simulink subsystem "Subsystem_Driver_Controllers_BAv01"  (R2022b)
settings: Solver=VariableStepAuto  StartTime=0.0  StopTime=10.0  RelTol=1e-3
undefined symbols (not defined in the file): param
libraries: slpidlib x2
settings Model: Creator=giaco  LastModifiedBy=giaco

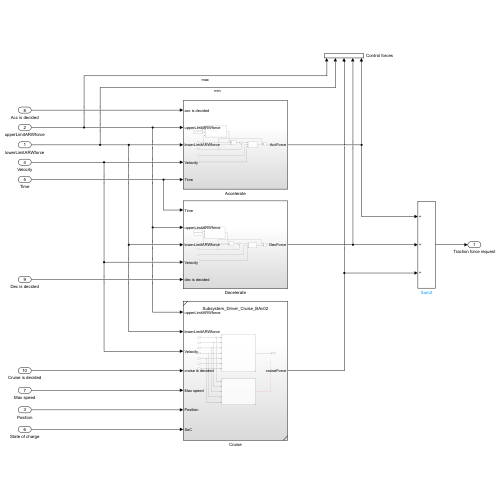
[thumbnail: Simulink's stored preview of the top-level diagram]
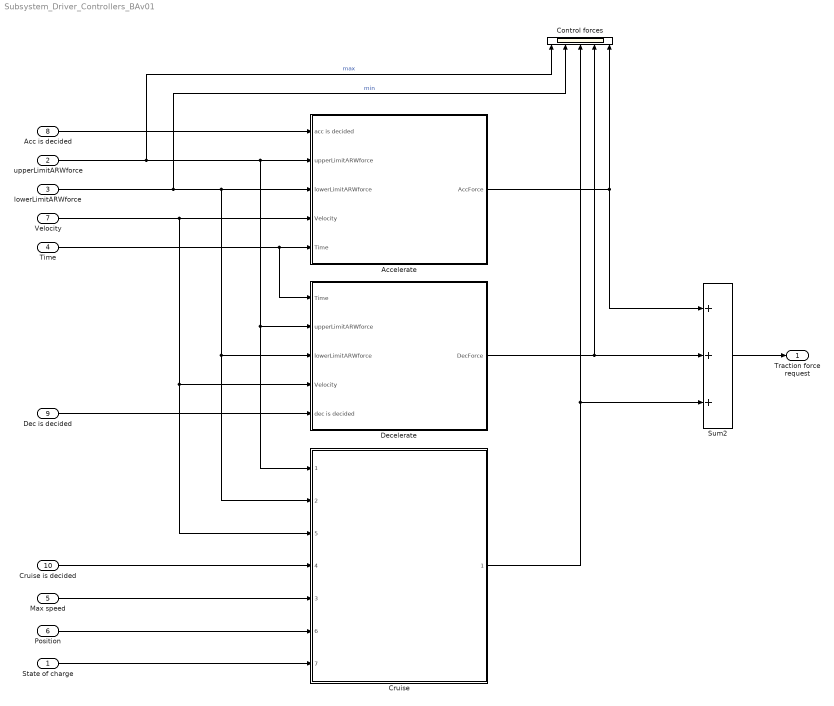
== system Subsystem_Driver_Controllers_BAv01 ==
  State of charge : Inport
  upperLimitARWforce : Inport  Port=2
  lowerLimitARWforce : Inport  Port=3
  Time : Inport  Port=4
  Max speed : Inport  Port=5
  Position : Inport  Port=6
  Velocity : Inport  Port=7
  Acc is decided : Inport  Port=8
  Dec is decided : Inport  Port=9
  Cruise is decided : Inport  Port=10
  Accelerate : Subsystem
  Control forces : Scope  NumInputPorts=5
  Cruise : Subsystem  ReferencedSubsystem=Subsystem_Driver_Cruise_BAv02
      settings: PortSchema="{\"entries\":[{\"content\":{\"sides\":[{\"content\":{\"connectorIds\":[\"In1\",\"In2\",\"In5\",\"In4\",\"In3\",\"In6\",\"In7\"]},\"type\":\"ConnectorPlacement.EquallySpacedRectSide\",\"uuid\":\"ef64809f-0964-4d4c-8634-68fa8e631720\"},{\"content\":{\"connectorIds\":[\"Out1\"],\"side\":\"RIGHT\"},\"type\":\"ConnectorPlacement.EquallySpacedRectSide\",\"uuid\":\"1cbe557a-e7d2-4fe5-a45b-503b50ba40bd\"},{\"content\":{\"connectorIds\":[],\"side\":\"TOP\"},\"type\":\"ConnectorPlacement.EquallySpacedRectSide\",\"uuid\":\"3b2eda76-9c7f-491f-ad4d-397cb13a64b5\"}]},\"type\":\"ConnectorPlacement.EquallySpacedConnector\",\"uuid\":\"83c1d113-dee0-4e25-92c9-f13a92a06a93\"}],\"packageUris\":[\"http://schema.mathworks.com/mf0/Connector/R2020b\"],\"version\":\"1.0\"}"
  Decelerate : Subsystem
  Sum2 : Sum  Inputs=+++
  Traction force request : Outport
  wires:
  upperLimitARWforce/1 -> Control forces/1, Accelerate/2(upperLimitARWforce), Decelerate/2(upperLimitARWforce), Cruise/1  "max"
  Max speed/1 -> Cruise/3
  Acc is decided/1 -> Accelerate/1(acc is decided)
  Accelerate/1(AccForce) -> Control forces/5, Sum2/1
  lowerLimitARWforce/1 -> Accelerate/3(lowerLimitARWforce), Decelerate/3(lowerLimitARWforce), Cruise/2, Control forces/2  "min"
  Sum2/1 -> Traction force request/1
  Decelerate/1(DecForce) -> Sum2/2, Control forces/4
  Time/1 -> Accelerate/5(Time), Decelerate/1(Time)
  State of charge/1 -> Cruise/7
  Dec is decided/1 -> Decelerate/5(dec is decided)
  Cruise/1 -> Control forces/3, Sum2/3
  Position/1 -> Cruise/6
  Cruise is decided/1 -> Cruise/4
  Velocity/1 -> Accelerate/4(Velocity), Decelerate/4(Velocity), Cruise/5

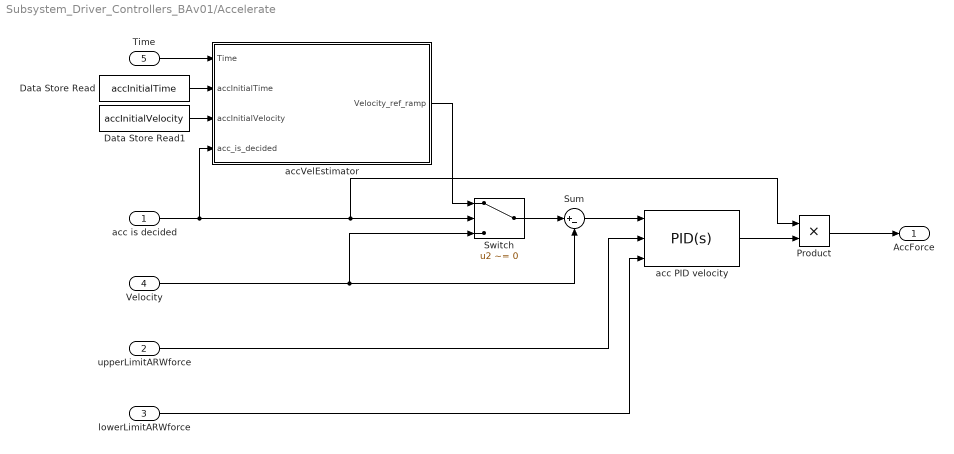
== system Subsystem_Driver_Controllers_BAv01/Accelerate ==
  acc is decided : Inport
  upperLimitARWforce : Inport  Port=2
  lowerLimitARWforce : Inport  Port=3
  Velocity : Inport  Port=4
  Time : Inport  Port=5
  Data Store Read : DataStoreRead  DataStoreName=accInitialTime  IndexOptions=Index vector (dialog)  Indices=1  OutputSizes=1
  Data Store Read1 : DataStoreRead  DataStoreName=accInitialVelocity  IndexOptions=Index vector (dialog)  Indices=1  OutputSizes=1
  Product : Product
  Sum : Sum  Inputs=|+-
  Switch : Switch  Criteria=u2 ~= 0  SaturateOnIntegerOverflow=off  InputSameDT=off
  acc PID velocity : slpidlib/PID Controller  Controller=PID  Form=Ideal  TimeDomain=Continuous-time  UseExternalTs=off  SampleTime=-1  IntegratorMethod=Forward Euler  FilterMethod=Forward Euler  ControllerParametersSource=internal  P=4000  I=1/(1/80)  UseKiTs=off  D=0  N=100  UseFilter=on  TunerSelectOption=Transfer Function Based (PID Tuner App)  InitialConditionSource=internal  InitialConditionForIntegrator=0  InitialConditionForFilter=0  DifferentiatorICPrevScaledInput=0  ExternalReset=none  TrackingMode=off  Kt=1  LimitOutput=on  SatLimitsSource=external  UpperSaturationLimit=param.motor.maxTorque * param.motor.transmissionRatio / param.suspension.wheelRadius  LowerSaturationLimit=param.motor.minTorque * param.motor.transmissionRatio / param.suspension.wheelRadius  LinearizeAsGain=on  AntiWindupMode=clamping  Kb=1  LimitIntegrator=off  UpperIntegratorSaturationLimit=inf  LowerIntegratorSaturationLimit=-inf  POutMin=[]  POutMax=[]  IOutMin=[]  IOutMax=[]  DOutMin=[]  DOutMax=[]  NOutMin=[]  NOutMax=[]  SumOutMin=[]  SumOutMax=[]  SaturationOutMin=[]  SaturationOutMax=[]  PParamMin=[]  PParamMax=[]  IParamMin=[]  IParamMax=[]  DParamMin=[]  DParamMax=[]  NParamMin=[]  NParamMax=[]  KbParamMin=[]  KbParamMax=[]  KtParamMin=[]  KtParamMax=[]  KbOutMin=[]  KbOutMax=[]  KtOutMin=[]  KtOutMax=[]  IntegratorOutMin=[]  IntegratorOutMax=[]  FilterOutMin=[]  FilterOutMax=[]  SumI1OutMin=[]  SumI1OutMax=[]  SumI2OutMin=[]  SumI2OutMax=[]  SumI3OutMin=[]  SumI3OutMax=[]  SumI4OutMin=[]  SumI4OutMax=[]  SumDOutMin=[]  SumDOutMax=[]  DifferentiatorOutMin=[]  DifferentiatorOutMax=[]  FilterDiffOutCoefMin=[]  FilterDiffOutCoefMax=[]  ReciprocalOutMin=[]  ReciprocalOutMax=[]  SumDenOutMin=[]  SumDenOutMax=[]  SumNumOutMin=[]  SumNumOutMax=[]  DivideOutMin=[]  DivideOutMax=[]  UdiffTsProdOutMin=[]  UdiffTsProdOutMax=[]  NTsProdOutMin=[]  NTsProdOutMax=[]  UintegralTsProdOutMin=[]  UintegralTsProdOutMax=[]  UngainTsProdOutMin=[]  UngainTsProdOutMax=[]  ClampingZeroOutDataTypeStr=Inherit: Inherit via back propagation  ClampingZeroOutMin=[]  ClampingZeroOutMax=[]  FilterDenConstantOutDataTypeStr=Inherit: Inherit via back propagation  FilterDenConstantOutMin=[]  FilterDenConstantOutMax=[]  PCopyOutDataTypeStr=Inherit: Inherit via back propagation  PCopyOutMin=[]  PCopyOutMax=[]  NCopyOutDataTypeStr=Inherit: Inherit via back propagation  NCopyOutMin=[]  NCopyOutMax=[]  IntegratorContinuousStateAttributes=''  IntegratorStateMustResolveToSignalObject=off  IntegratorRTWStateStorageClass=Auto  FilterContinuousStateAttributes=''  FilterStateMustResolveToSignalObject=off  FilterRTWStateStorageClass=Auto  ParallelPVariant=Passthrough  IdealPVariant=InternalParameters  IVariant=InternalParameters  DVariant=InternalParameters  IntegratorVariant=Continuous  SatVariant=External  AWVariant=ContClampingIdeal  PCopyVariant=InternalParamsIdeal  TRVariant=Disabled  FdbkBlocksVariant=Forward  IdealPFdbkVariant=Disabled  SatFdbkVariant=Disabled  DerivativeFilterVariant=ContFilter  NVariant=InternalParameters  NCopyVariant=Disabled  FilterICVariant=InternalICsFilter  IntegratorICVariant=InternalICs  ExternalResetVariant=Disabled  TRSumVariant=Passthrough  SumFdbkVariant=Disabled  SumVariant=Sum_PID  TsampFilterVariant=InternalTs  TsampNgainVariant=Passthrough  TsampIntegralVariant=Passthrough  ExternalSaturationOutDataTypeStr=Inherit: Same as second input
  accVelEstimator : MATLAB Function  TreatAsAtomicUnit=on
  AccForce : Outport
  wires:
  acc is decided/1 -> accVelEstimator/4(acc_is_decided), Product/1, Switch/2
  Switch/1 -> Sum/1
  Velocity/1 -> Sum/2, Switch/3
  Sum/1 -> acc PID velocity/1
  acc PID velocity/1 -> Product/2
  Product/1 -> AccForce/1
  Time/1 -> accVelEstimator/1(Time)
  accVelEstimator/1(Velocity_ref_ramp) -> Switch/1
  Data Store Read/1 -> accVelEstimator/2(accInitialTime)
  Data Store Read1/1 -> accVelEstimator/3(accInitialVelocity)
  upperLimitARWforce/1 -> acc PID velocity/2
  lowerLimitARWforce/1 -> acc PID velocity/3

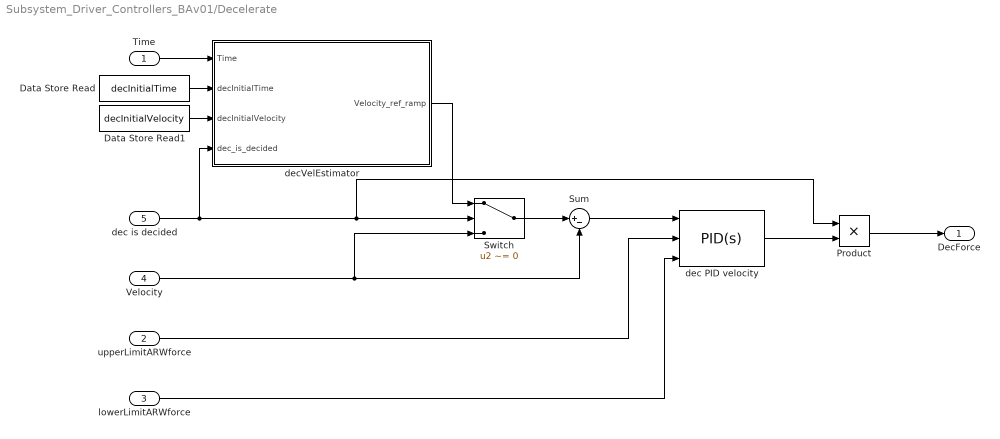
== system Subsystem_Driver_Controllers_BAv01/Decelerate ==
  Time : Inport
  upperLimitARWforce : Inport  Port=2
  lowerLimitARWforce : Inport  Port=3
  Velocity : Inport  Port=4
  dec is decided : Inport  Port=5
  Data Store Read : DataStoreRead  DataStoreName=decInitialTime  IndexOptions=Index vector (dialog)  Indices=1  OutputSizes=1
  Data Store Read1 : DataStoreRead  DataStoreName=decInitialVelocity  IndexOptions=Index vector (dialog)  Indices=1  OutputSizes=1
  Product : Product
  Sum : Sum  Inputs=|+-
  Switch : Switch  Criteria=u2 ~= 0  SaturateOnIntegerOverflow=off  InputSameDT=off
  dec PID velocity : slpidlib/PID Controller  Controller=PID  Form=Ideal  TimeDomain=Continuous-time  UseExternalTs=off  SampleTime=-1  IntegratorMethod=Forward Euler  FilterMethod=Forward Euler  ControllerParametersSource=internal  P=4000  I=1/(1/80)  UseKiTs=off  D=0  N=100  UseFilter=on  TunerSelectOption=Transfer Function Based (PID Tuner App)  InitialConditionSource=internal  InitialConditionForIntegrator=0  InitialConditionForFilter=0  DifferentiatorICPrevScaledInput=0  ExternalReset=none  TrackingMode=off  Kt=1  LimitOutput=on  SatLimitsSource=external  UpperSaturationLimit=param.motor.maxTorque * param.motor.transmissionRatio / param.suspension.wheelRadius  LowerSaturationLimit=param.motor.minTorque * param.motor.transmissionRatio / param.suspension.wheelRadius  LinearizeAsGain=on  AntiWindupMode=clamping  Kb=1  LimitIntegrator=off  UpperIntegratorSaturationLimit=inf  LowerIntegratorSaturationLimit=-inf  POutMin=[]  POutMax=[]  IOutMin=[]  IOutMax=[]  DOutMin=[]  DOutMax=[]  NOutMin=[]  NOutMax=[]  SumOutMin=[]  SumOutMax=[]  SaturationOutMin=[]  SaturationOutMax=[]  PParamMin=[]  PParamMax=[]  IParamMin=[]  IParamMax=[]  DParamMin=[]  DParamMax=[]  NParamMin=[]  NParamMax=[]  KbParamMin=[]  KbParamMax=[]  KtParamMin=[]  KtParamMax=[]  KbOutMin=[]  KbOutMax=[]  KtOutMin=[]  KtOutMax=[]  IntegratorOutMin=[]  IntegratorOutMax=[]  FilterOutMin=[]  FilterOutMax=[]  SumI1OutMin=[]  SumI1OutMax=[]  SumI2OutMin=[]  SumI2OutMax=[]  SumI3OutMin=[]  SumI3OutMax=[]  SumI4OutMin=[]  SumI4OutMax=[]  SumDOutMin=[]  SumDOutMax=[]  DifferentiatorOutMin=[]  DifferentiatorOutMax=[]  FilterDiffOutCoefMin=[]  FilterDiffOutCoefMax=[]  ReciprocalOutMin=[]  ReciprocalOutMax=[]  SumDenOutMin=[]  SumDenOutMax=[]  SumNumOutMin=[]  SumNumOutMax=[]  DivideOutMin=[]  DivideOutMax=[]  UdiffTsProdOutMin=[]  UdiffTsProdOutMax=[]  NTsProdOutMin=[]  NTsProdOutMax=[]  UintegralTsProdOutMin=[]  UintegralTsProdOutMax=[]  UngainTsProdOutMin=[]  UngainTsProdOutMax=[]  ClampingZeroOutDataTypeStr=Inherit: Inherit via back propagation  ClampingZeroOutMin=[]  ClampingZeroOutMax=[]  FilterDenConstantOutDataTypeStr=Inherit: Inherit via back propagation  FilterDenConstantOutMin=[]  FilterDenConstantOutMax=[]  PCopyOutDataTypeStr=Inherit: Inherit via back propagation  PCopyOutMin=[]  PCopyOutMax=[]  NCopyOutDataTypeStr=Inherit: Inherit via back propagation  NCopyOutMin=[]  NCopyOutMax=[]  IntegratorContinuousStateAttributes=''  IntegratorStateMustResolveToSignalObject=off  IntegratorRTWStateStorageClass=Auto  FilterContinuousStateAttributes=''  FilterStateMustResolveToSignalObject=off  FilterRTWStateStorageClass=Auto  ParallelPVariant=Passthrough  IdealPVariant=InternalParameters  IVariant=InternalParameters  DVariant=InternalParameters  IntegratorVariant=Continuous  SatVariant=External  AWVariant=ContClampingIdeal  PCopyVariant=InternalParamsIdeal  TRVariant=Disabled  FdbkBlocksVariant=Forward  IdealPFdbkVariant=Disabled  SatFdbkVariant=Disabled  DerivativeFilterVariant=ContFilter  NVariant=InternalParameters  NCopyVariant=Disabled  FilterICVariant=InternalICsFilter  IntegratorICVariant=InternalICs  ExternalResetVariant=Disabled  TRSumVariant=Passthrough  SumFdbkVariant=Disabled  SumVariant=Sum_PID  TsampFilterVariant=InternalTs  TsampNgainVariant=Passthrough  TsampIntegralVariant=Passthrough  ExternalSaturationOutDataTypeStr=Inherit: Same as second input
  decVelEstimator : MATLAB Function  TreatAsAtomicUnit=on
  DecForce : Outport
  wires:
  dec is decided/1 -> decVelEstimator/4(dec_is_decided), Product/1, Switch/2
  Switch/1 -> Sum/1
  Velocity/1 -> Sum/2, Switch/3
  dec PID velocity/1 -> Product/2
  Sum/1 -> dec PID velocity/1
  Product/1 -> DecForce/1
  Time/1 -> decVelEstimator/1(Time)
  Data Store Read1/1 -> decVelEstimator/3(decInitialVelocity)
  decVelEstimator/1(Velocity_ref_ramp) -> Switch/1
  Data Store Read/1 -> decVelEstimator/2(decInitialTime)
  upperLimitARWforce/1 -> dec PID velocity/2
  lowerLimitARWforce/1 -> dec PID velocity/3

== matlab function Subsystem_Driver_Controllers_BAv01/Accelerate/accVelEstimator ==
  data: Time input; Velocity_ref_ramp output; accInitialTime input; accInitialVelocity input; driver parameter; acc_is_decided input
function Velocity_ref_ramp = accVelEstimator(Time, accInitialTime, accInitialVelocity, driver, acc_is_decided)

Velocity_ref_ramp = 0;

if acc_is_decided
    Velocity_ref_ramp = driver.accRef .* (Time - accInitialTime) + accInitialVelocity;
end

== matlab function Subsystem_Driver_Controllers_BAv01/Decelerate/decVelEstimator ==
  data: Time input; Velocity_ref_ramp output; decInitialTime input; decInitialVelocity input; driver parameter; dec_is_decided input
function Velocity_ref_ramp = decVelEstimator(Time, decInitialTime, decInitialVelocity, driver, dec_is_decided)

Velocity_ref_ramp = 0;

if dec_is_decided
    Velocity_ref_ramp = driver.decRef .* (Time - decInitialTime) + decInitialVelocity;
end
